simulink model "SVPWM3"  (R2020a)
settings: Solver=ode23s  StartTime=0.0  StopTime=0.1  MaxStep=0.00001  RelTol=1e-6
libraries: simulink x1
settings Model: Creator=heliang  LastModifiedBy=heliang

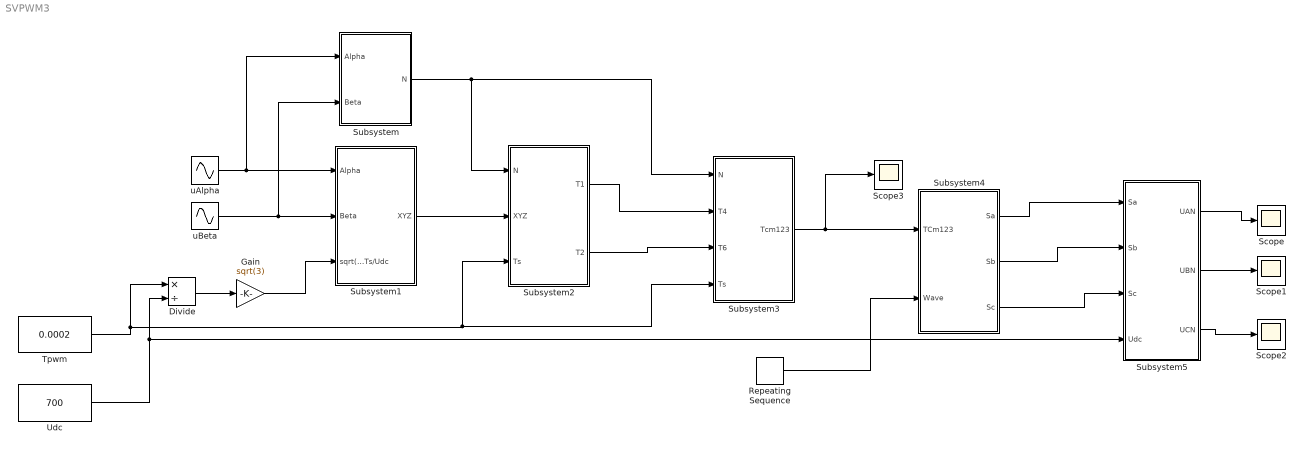
== system SVPWM3 ==
  Divide : Product  Inputs=*/
  Gain : Gain  Gain=sqrt(3)
  Repeating Sequence : simulink/Sources/Repeating Sequence  rep_seq_t=[0 1/10000 1/5000]  rep_seq_y=[0 1/10000 0]
  Scope{,1..3} (4 alike) : Scope
  Subsystem : Subsystem
  Subsystem1 : Subsystem
  Subsystem2 : Subsystem
  Subsystem3 : Subsystem
  Subsystem4 : Subsystem
  Subsystem5 : Subsystem
  Tpwm : Constant  Value=0.0002
  Udc : Constant  Value=700
  uAlpha : Sin  Amplitude=200  Frequency=2*50*pi  SampleTime=0
  uBeta : Sin  Amplitude=200  Frequency=100*pi  Phase=pi/2  SampleTime=0
  wires:
  Tpwm/1 -> Subsystem3/4(Ts), Subsystem2/3(Ts), Divide/1
  Udc/1 -> Subsystem5/4(Udc), Divide/2
  Divide/1 -> Gain/1
  Gain/1 -> Subsystem1/3(sqrt(3)*Ts/Udc)
  uBeta/1 -> Subsystem/2(Beta), Subsystem1/2(Beta)
  uAlpha/1 -> Subsystem/1("Alpha "), Subsystem1/1("Alpha ")
  Subsystem/1(N) -> Subsystem3/1(N), Subsystem2/1(N)
  Subsystem1/1(XYZ) -> Subsystem2/2("XYZ ")
  Subsystem2/1(T1) -> Subsystem3/2(T4)
  Subsystem2/2(T2) -> Subsystem3/3(T6)
  Subsystem3/1(Tcm123) -> Scope3/1, Subsystem4/1(TCm123)
  Repeating Sequence/1 -> Subsystem4/2(Wave)
  Subsystem4/1(Sa) -> Subsystem5/1(Sa)
  Subsystem4/2(Sb) -> Subsystem5/2(Sb)
  Subsystem4/3(Sc) -> Subsystem5/3(Sc)
  Subsystem5/1(UAN) -> Scope/1
  Subsystem5/2(UBN) -> Scope1/1
  Subsystem5/3(UCN) -> Scope2/1

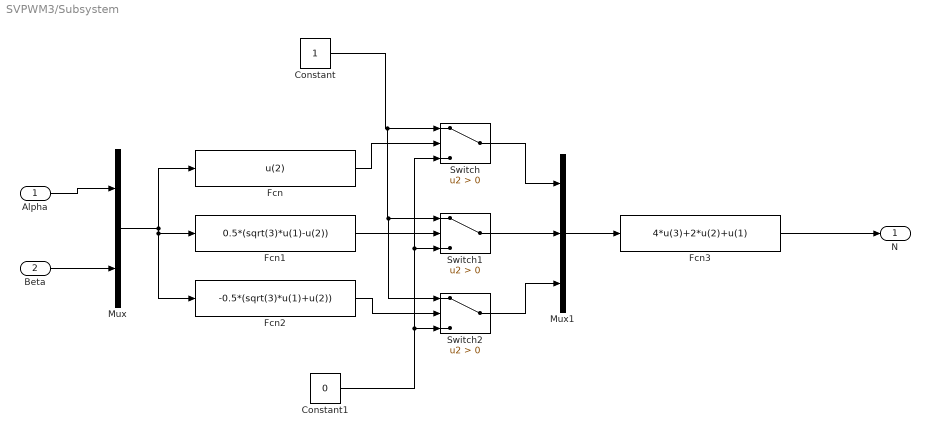
== system SVPWM3/Subsystem ==
  "Alpha " : Inport
  Beta : Inport  Port=2
  Constant : Constant
  Constant1 : Constant  Value=0
  Fcn : Fcn  Expr=u(2)
  Fcn1 : Fcn  Expr=0.5*(sqrt(3)*u(1)-u(2))
  Fcn2 : Fcn  Expr=-0.5*(sqrt(3)*u(1)+u(2))
  Fcn3 : Fcn  Expr=4*u(3)+2*u(2)+u(1)
  Mux : Mux  Inputs=2
  Mux1 : Mux  Inputs=3
  Switch : Switch  Criteria=u2 > Threshold
  Switch1 : Switch  Criteria=u2 > Threshold
  Switch2 : Switch  Criteria=u2 > Threshold
  N : Outport
  wires:
  Beta/1 -> Mux/2
  "Alpha "/1 -> Mux/1
  Mux/1 -> Fcn2/1, Fcn1/1, Fcn/1
  Constant/1 -> Switch2/1, Switch1/1, Switch/1
  Constant1/1 -> Switch2/3, Switch1/3, Switch/3
  Fcn/1 -> Switch/2
  Fcn1/1 -> Switch1/2
  Fcn2/1 -> Switch2/2
  Switch/1 -> Mux1/1
  Switch1/1 -> Mux1/2
  Switch2/1 -> Mux1/3
  Mux1/1 -> Fcn3/1
  Fcn3/1 -> N/1

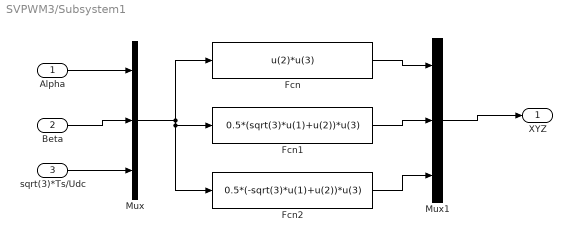
== system SVPWM3/Subsystem1 ==
  "Alpha " : Inport
  Beta : Inport  Port=2
  sqrt(3)*Ts/Udc : Inport  Port=3
  Fcn : Fcn  Expr=u(2)*u(3)
  Fcn1 : Fcn  Expr=0.5*(sqrt(3)*u(1)+u(2))*u(3)
  Fcn2 : Fcn  Expr=0.5*(-sqrt(3)*u(1)+u(2))*u(3)
  Mux : Mux  Inputs=3
  Mux1 : Mux  Inputs=3
  XYZ : Outport
  wires:
  Mux/1 -> Fcn/1, Fcn1/1, Fcn2/1
  "Alpha "/1 -> Mux/1
  Beta/1 -> Mux/2
  sqrt(3)*Ts/Udc/1 -> Mux/3
  Fcn/1 -> Mux1/1
  Fcn1/1 -> Mux1/2
  Fcn2/1 -> Mux1/3
  Mux1/1 -> XYZ/1

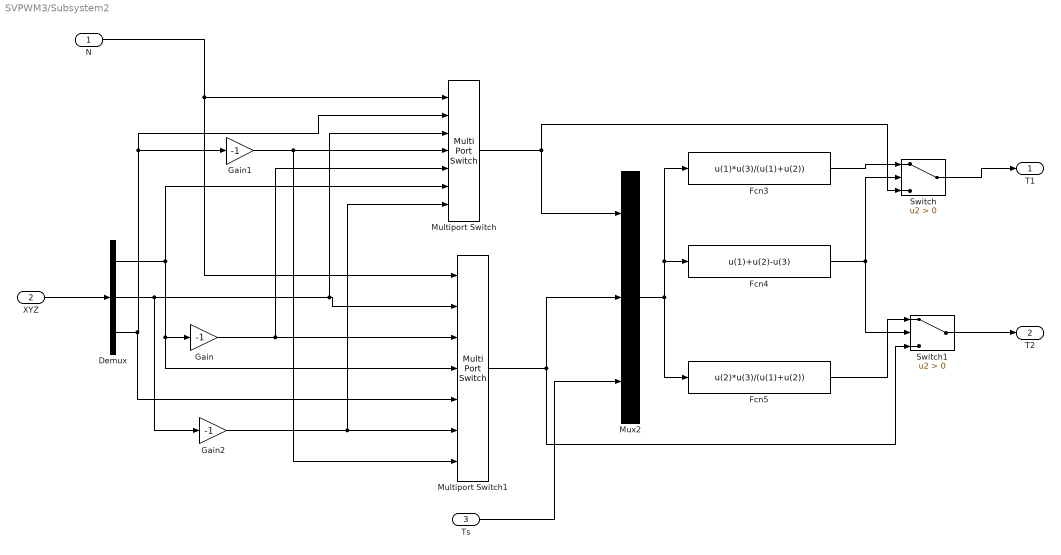
== system SVPWM3/Subsystem2 ==
  N : Inport
  "XYZ " : Inport  Port=2
  Ts : Inport  Port=3
  Demux : Demux  Outputs=3
  Fcn3 : Fcn  Expr=u(1)*u(3)/(u(1)+u(2))
  Fcn4 : Fcn  Expr=u(1)+u(2)-u(3)
  Fcn5 : Fcn  Expr=u(2)*u(3)/(u(1)+u(2))
  Gain : Gain  Gain=-1
  Gain1 : Gain  Gain=-1
  Gain2 : Gain  Gain=-1
  Multiport Switch : MultiPortSwitch  Inputs=6
  Multiport Switch1 : MultiPortSwitch  Inputs=6
  Mux2 : Mux  Inputs=3
  Switch : Switch  Criteria=u2 > Threshold
  Switch1 : Switch  Criteria=u2 > Threshold
  T1 : Outport
  T2 : Outport  Port=2
  wires:
  "XYZ "/1 -> Demux/1
  N/1 -> Multiport Switch/1, Multiport Switch1/1
  Demux/2 -> Gain2/1, Multiport Switch/3, Multiport Switch1/2
  Gain/1 -> Multiport Switch/5, Multiport Switch1/3
  Demux/1 -> Multiport Switch1/4, Gain/1, Multiport Switch/6
  Gain1/1 -> Multiport Switch1/7, Multiport Switch/4
  Demux/3 -> Multiport Switch1/5, Gain1/1, Multiport Switch/2
  Gain2/1 -> Multiport Switch/7, Multiport Switch1/6
  Multiport Switch/1 -> Mux2/1, Switch/3
  Multiport Switch1/1 -> Mux2/2, Switch1/3
  Ts/1 -> Mux2/3
  Mux2/1 -> Fcn5/1, Fcn4/1, Fcn3/1
  Fcn4/1 -> Switch/2, Switch1/2
  Fcn3/1 -> Switch/1
  Fcn5/1 -> Switch1/1
  Switch1/1 -> T2/1
  Switch/1 -> T1/1

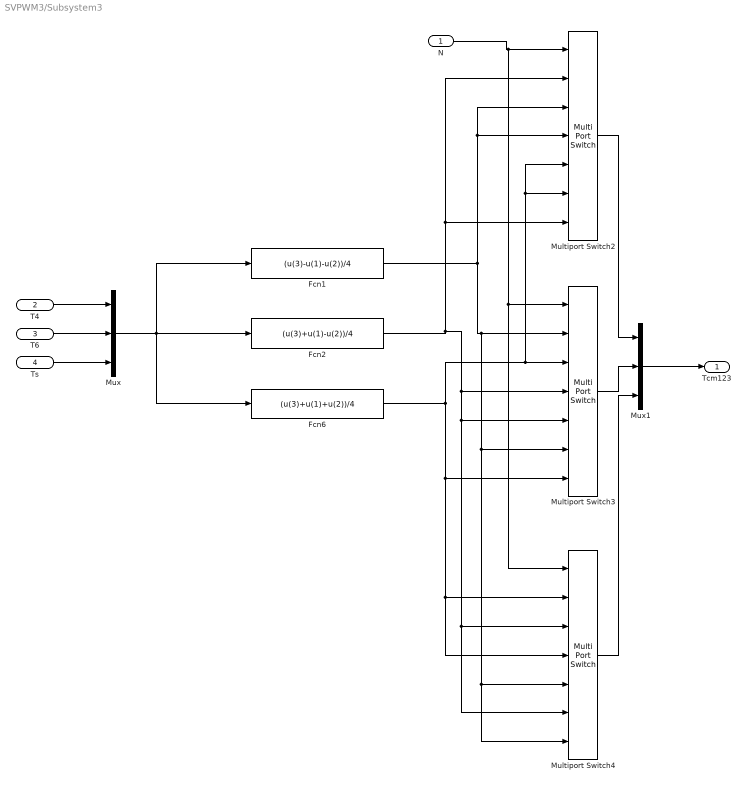
== system SVPWM3/Subsystem3 ==
  N : Inport
  T4 : Inport  Port=2
  T6 : Inport  Port=3
  Ts : Inport  Port=4
  Fcn1 : Fcn  Expr=(u(3)-u(1)-u(2))/4
  Fcn2 : Fcn  Expr=(u(3)+u(1)-u(2))/4
  Fcn6 : Fcn  Expr=(u(3)+u(1)+u(2))/4
  Multiport Switch2 : MultiPortSwitch  Inputs=6
  Multiport Switch3 : MultiPortSwitch  Inputs=6
  Multiport Switch4 : MultiPortSwitch  Inputs=6
  Mux : Mux  Inputs=3
  Mux1 : Mux  Inputs=3
  Tcm123 : Outport
  wires:
  Mux/1 -> Fcn1/1, Fcn6/1, Fcn2/1
  N/1 -> Multiport Switch4/1, Multiport Switch3/1, Multiport Switch2/1
  T4/1 -> Mux/1
  T6/1 -> Mux/2
  Ts/1 -> Mux/3
  Fcn2/1 -> Multiport Switch3/4, Multiport Switch3/5, Multiport Switch4/6, Multiport Switch4/3, Multiport Switch2/7, Multiport Switch2/2
  Fcn1/1 -> Multiport Switch3/6, Multiport Switch4/7, Multiport Switch4/5, Multiport Switch3/2, Multiport Switch2/4, Multiport Switch2/3
  Fcn6/1 -> Multiport Switch3/7, Multiport Switch4/4, Multiport Switch4/2, Multiport Switch2/6, Multiport Switch2/5, Multiport Switch3/3
  Multiport Switch2/1 -> Mux1/1
  Multiport Switch3/1 -> Mux1/2
  Multiport Switch4/1 -> Mux1/3
  Mux1/1 -> Tcm123/1

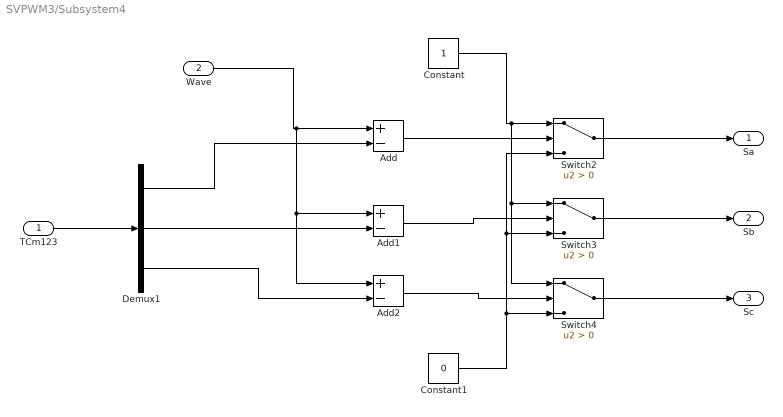
== system SVPWM3/Subsystem4 ==
  TCm123 : Inport
  Wave : Inport  Port=2
  Add : Sum  Inputs=+-
  Add1 : Sum  Inputs=+-
  Add2 : Sum  Inputs=+-
  Constant : Constant
  Constant1 : Constant  Value=0
  Demux1 : Demux  Outputs=3
  Switch2 : Switch  Criteria=u2 > Threshold
  Switch3 : Switch  Criteria=u2 > Threshold
  Switch4 : Switch  Criteria=u2 > Threshold
  Sa : Outport
  Sb : Outport  Port=2
  Sc : Outport  Port=3
  wires:
  Wave/1 -> Add2/1, Add1/1, Add/1
  TCm123/1 -> Demux1/1
  Demux1/1 -> Add/2
  Demux1/2 -> Add1/2
  Demux1/3 -> Add2/2
  Add/1 -> Switch2/2
  Add2/1 -> Switch4/2
  Add1/1 -> Switch3/2
  Constant/1 -> Switch4/1, Switch3/1, Switch2/1
  Constant1/1 -> Switch2/3, Switch3/3, Switch4/3
  Switch3/1 -> Sb/1
  Switch2/1 -> Sa/1
  Switch4/1 -> Sc/1

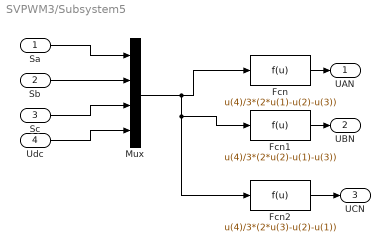
== system SVPWM3/Subsystem5 ==
  Sa : Inport
  Sb : Inport  Port=2
  Sc : Inport  Port=3
  Udc : Inport  Port=4
  Fcn : Fcn  Expr=u(4)/3*(2*u(1)-u(2)-u(3))
  Fcn1 : Fcn  Expr=u(4)/3*(2*u(2)-u(1)-u(3))
  Fcn2 : Fcn  Expr=u(4)/3*(2*u(3)-u(2)-u(1))
  Mux : Mux
  UAN : Outport
  UBN : Outport  Port=2
  UCN : Outport  Port=3
  wires:
  Sa/1 -> Mux/1
  Sb/1 -> Mux/2
  Fcn/1 -> UAN/1
  Sc/1 -> Mux/3
  Udc/1 -> Mux/4
  Mux/1 -> Fcn1/1, Fcn2/1, Fcn/1
  Fcn2/1 -> UCN/1
  Fcn1/1 -> UBN/1
